simulink model "Pole_placement"  (R2023b)
settings: Solver=VariableStepAuto  StartTime=0.0  StopTime=20  MaxStep=0.05  MinStep=0.001  RelTol=1e-3
values from neighbouring files (symbols this model uses):
  A = double(A)    [Rotational_inverted_pendulum.m]
  A_uns = double(A_uns)    [Rotational_inverted_pendulum.m]
  alfa = 1e-5    (= 1e-05)    [Rotational_inverted_pendulum.m]
  B = double(B)    [Rotational_inverted_pendulum.m]
  B_uns = double(B_uns)    [Rotational_inverted_pendulum.m]
  beta = 1.295e-5    (= 1.295e-05)    [Rotational_inverted_pendulum.m]
  C = [1 0 0 0 ... (first row only)    [Rotational_inverted_pendulum.m]
  C_uns = [1 0 0 0 ... (first row only)    [Rotational_inverted_pendulum.m]
  D = [0 ... (first row only)    [Rotational_inverted_pendulum.m]
  D_uns = [0 ... (first row only)    [Rotational_inverted_pendulum.m]
  g0 = 9.81    [Rotational_inverted_pendulum.m]
  Ip = (mp*Lp^2)/12    (= 3.3282e-05)    [Rotational_inverted_pendulum.m]
  Ir = 9.6e-5    (= 9.6e-05)    [Rotational_inverted_pendulum.m]
  Ir_tot = Ir+J+J_hub    (= 0.0001006)    [Rotational_inverted_pendulum.m]
  K = 42e-3    (= 0.042)    [Rotational_inverted_pendulum.m]
  K_pp = place(A,B,P)    [Rotational_inverted_pendulum.m]
  K_pp_uns = place(A_uns,B_uns,P_uns)    [Rotational_inverted_pendulum.m]
  L_kf = lqr(A',C',Q_tilde,R_tilde)'    [Rotational_inverted_pendulum.m]
  L_kf_uns = lqr(A_uns',C_uns',Q_tilde_uns,R_tilde_uns)'    [Rotational_inverted_pendulum.m]
  L_pp = place(A',C',P_obsv)'    [Rotational_inverted_pendulum.m]
  L_pp_uns = place(A_uns',C_uns',P_obsv_uns)'    [Rotational_inverted_pendulum.m]
  La = 1.16e-3    (= 0.00116)    [Rotational_inverted_pendulum.m]
  Ld = 0.40*Lr    (= 0.034)    [Rotational_inverted_pendulum.m]
  Lp = 0.129    [Rotational_inverted_pendulum.m]
  Lr = 0.085    [Rotational_inverted_pendulum.m]
  mp = 0.024    [Rotational_inverted_pendulum.m]
  mr = 0.095    [Rotational_inverted_pendulum.m]
  phi_dot_init = 0    [Rotational_inverted_pendulum.m]
  phi_init = 0    [Rotational_inverted_pendulum.m]
  Ra = 8.4    [Rotational_inverted_pendulum.m]
  theta_dot_init = 0    [Rotational_inverted_pendulum.m]
  theta_init = 0    [Rotational_inverted_pendulum.m]
  x1_bar = double(sol.x1)    [Rotational_inverted_pendulum.m]
  x1_bar_uns = x1_bar    [Rotational_inverted_pendulum.m]
  x3_bar = 0    [Rotational_inverted_pendulum.m]
  x3_bar_uns = pi    (= 3.14159265359)    [Rotational_inverted_pendulum.m]
undefined symbols (not defined in the file or in its folder): rot_pend
libraries: simulink_extras x17
settings Model: Creator=Mark  LastModifiedBy=Mark

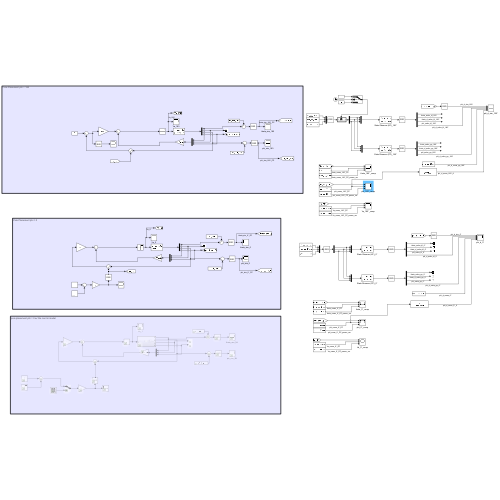
[thumbnail: Simulink's stored preview of the top-level diagram]
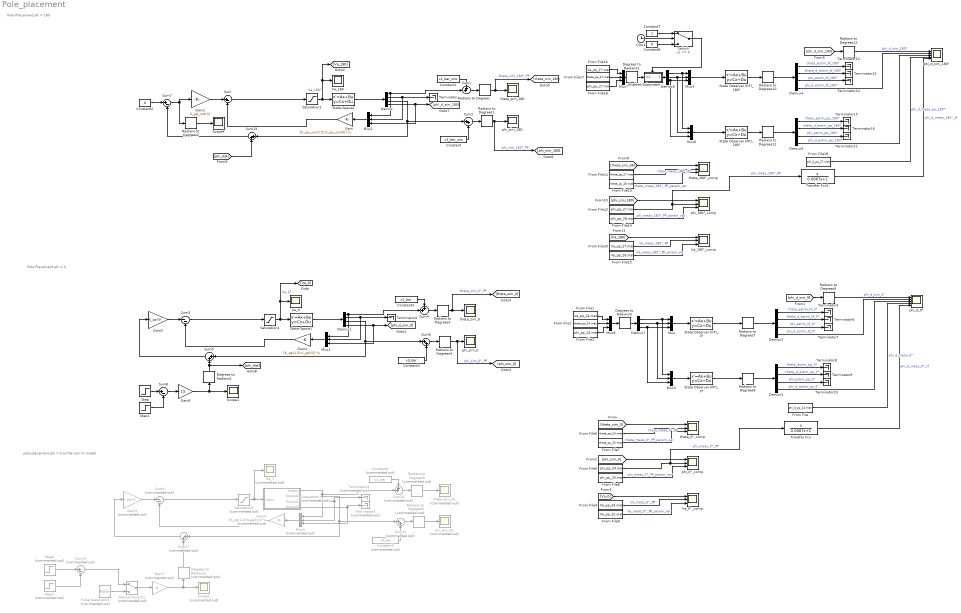
== system Pole_placement ==
  note: pole placement phi = 0 w/ the non lin model
  note: Pole Placement phi = 180
  note: Pole Placement phi = 0
  Clock : Clock
  Constant : Constant  Value=x3_bar_uns
  Constant1 : Constant  Value=x1_bar_uns
  Constant2 : Constant  Value=0
  Constant3 : Constant  Value=x3_bar
  Constant4 : Constant  Value=x1_bar
  Constant5 : Constant  Commented=on  Value=x3_bar
  Constant6 : Constant  Commented=on  Value=x1_bar
  Constant7 : Constant
  Constant8 : Constant  Value=0
  Degrees to Radians1 : simulink_extras/Transformations/Degrees to Radians
  Degrees to Radians2 : simulink_extras/Transformations/Degrees to Radians  Commented=on
  Degrees to Radians3 : simulink_extras/Transformations/Degrees to Radians
  Degrees to Radians4 : simulink_extras/Transformations/Degrees to Radians
  Demux{,1..5} (6 alike) : Demux
  Demux6 : Demux  Outputs=3
  Demux7 : Demux  Outputs=3
  Enabled Subsystem : Subsystem  TreatAsAtomicUnit=on
  From File : FromFile  FileName=phi_d_pp_24.mat  SampleTime=0
  From File1 : FromFile  FileName=Va_pp_24.mat  SampleTime=0
  From File10 : FromFile  FileName=Va_pp_27.mat  SampleTime=0
  From File11 : FromFile  FileName=theta_pp_27.mat  SampleTime=0
  From File12 : FromFile  FileName=phi_pp_27.mat  SampleTime=0
  From File13 : FromFile  FileName=theta_pp_28.mat  SampleTime=0
  From File14 : FromFile  FileName=phi_pp_28.mat  SampleTime=0
  From File15 : FromFile  FileName=Va_pp_28.mat  SampleTime=0
  From File16 : FromFile  FileName=Va_pp_27.mat  SampleTime=0
  From File17 : FromFile  FileName=theta_pp_27.mat  SampleTime=0
  From File18 : FromFile  FileName=phi_pp_27.mat  SampleTime=0
  From File19 : FromFile  FileName=phi_d_pp_27.mat  SampleTime=0
  From File2 : FromFile  FileName=theta_pp_24.mat  SampleTime=0
  From File3 : FromFile  FileName=phi_pp_24.mat  SampleTime=0
  From File4 : FromFile  FileName=Va_pp_24.mat  SampleTime=0
  From File5 : FromFile  FileName=theta_pp_24.mat  SampleTime=0
  From File6 : FromFile  FileName=phi_pp_24.mat  SampleTime=0
  From File7 : FromFile  FileName=theta_pp_25.mat  SampleTime=0
  From File8 : FromFile  FileName=phi_pp_25.mat  SampleTime=0
  From File9 : FromFile  FileName=Va_pp_25.mat  SampleTime=0
  Gain : Gain  Gain=[K_pp_uns(1:2) K_pp_uns(4)]  Multiplication=Matrix(K*u) (u vector)
  Gain1 : Gain  Gain=K_pp_uns(3)
  Gain2 : Gain  Gain=[K_pp(1:2) K_pp(4)]  Multiplication=Matrix(K*u) (u vector)
  Gain3 : Gain  Gain=K_pp(3)
  Gain4 : Gain  Commented=on  Gain=[K_pp(1:2) K_pp(4)]  Multiplication=Matrix(K*u) (u vector)
  Gain5 : Gain  Commented=on  Gain=K_pp(3)
  Gain6 : Gain  Gain=15
  Gain7 : Gain  Commented=on  Gain=5
  Manual Switch1 : ManualSwitch  Commented=on
  Mux{,1..2,4..8} (8 alike) : Mux  Inputs=3
  Mux3 : Mux  Commented=on  Inputs=3
  Pulse Generator2 : DiscretePulseGenerator  Commented=on  PulseType=Time based  Period=10000  PulseWidth=0.005  PhaseDelay=30
  Radians to Degrees{,1..4,7..12} (11 alike) : simulink_extras/Transformations/Radians to Degrees
  Radians to Degrees5 : simulink_extras/Transformations/Radians to Degrees  Commented=on
  Radians to Degrees6 : simulink_extras/Transformations/Radians to Degrees  Commented=on
  Saturation1 : Saturate  UpperLimit=10  LowerLimit=-10
  Saturation2 : Saturate  UpperLimit=10  LowerLimit=-10
  Saturation3 : Saturate  Commented=on  UpperLimit=10  LowerLimit=-10
  Scope1 : Scope
  Scope2 : Scope  Commented=on
  Scope4 : Scope
  State Observer (KF)_0° : StateSpace  A=A-L_kf*C  B=[B-L_kf*D L_kf]  C=eye(4)  D=zeros(4,3)  InitialCondition=0  ParameterTunability=Unconstrained
  State Observer (KF)_180° : StateSpace  A=A_uns-L_kf_uns*C_uns  B=[B_uns-L_kf_uns*D_uns L_kf_uns]  C=eye(4)  D=zeros(4,3)  InitialCondition=0  ParameterTunability=Unconstrained
  State Observer (PP)_0° : StateSpace  A=A-L_pp*C  B=[B-L_pp*D L_pp]  C=eye(4)  D=zeros(4,3)  InitialCondition=0
  State Observer (PP)_180° : StateSpace  A=A_uns-L_pp_uns*C_uns  B=[B_uns-L_pp_uns*D_uns L_pp_uns]  C=eye(4)  D=zeros(4,3)  InitialCondition=[0 0 0 0]
  State-Space1 : StateSpace  A=A  B=B  C=eye(4)  D=zeros(4,1)  InitialCondition=[0 0 0 0]
  State-Space2 : StateSpace  A=A_uns  B=B_uns  C=[1 0 0 0; 0 1 0 0; 0 0 1 0; 0 0 0 1]  D=[0 0 0 0]'  InitialCondition=[0 0 0 0]
  Step : Step  Time=10  SampleTime=0
  Step1 : Step  Time=10.05  SampleTime=0
  Step2 : Step  Commented=on  Time=30  SampleTime=0
  Step3 : Step  Commented=on  Time=30.05  SampleTime=0
  Subsystem1 : Subsystem  Commented=on
  Sum : Sum  Inputs=|+-
  Sum1 : Sum  Inputs=++|
  Sum10 : Sum  Commented=on  Inputs=++|
  Sum11 : Sum  Commented=on  Inputs=|++
  Sum12 : Sum  Commented=on  Inputs=|++
  Sum{2,5..6,13} (4 alike) : Sum  Inputs=|++
  Sum14 : Sum  Commented=on  Inputs=|+-
  Sum3 : Sum  Inputs=|--
  Sum4 : Sum  Inputs=++|
  Sum7 : Sum  Inputs=|+-
  Sum8 : Sum  Inputs=|+-
  Sum9 : Sum  Commented=on  Inputs=|--
  Switch : Switch  SaturateOnIntegerOverflow=off  InputSameDT=off
  Terminator{,2..3,6..16} (14 alike) : Terminator
  Terminator4 : Terminator  Commented=on
  Terminator5 : Terminator  Commented=on
  Transfer Fcn : TransferFcn  Numerator=[1 0]  Denominator=[0.0067 1]
  Transfer Fcn1 : TransferFcn  Numerator=[1 0]  Denominator=[0.0067 1]
  Va_0 : Scope
  Va_0°_comp : Scope  NumInputPorts=3
  Va_1 : Scope  Commented=on
  Va_180 : Scope
  Va_180°_comp : Scope  NumInputPorts=3
  phi_0°_comp : Scope  NumInputPorts=3
  phi_180°_comp : Scope  NumInputPorts=3
  phi_d_0° : Scope  NumInputPorts=5
  phi_d_sim_180° : Scope  NumInputPorts=5
  phi_sim_0 : Scope
  phi_sim_180 : Scope
  phi_sim_NL : Scope  Commented=on
  theta_0°_comp : Scope  NumInputPorts=3
  theta_180°_comp : Scope  NumInputPorts=3
  theta_sim_0 : Scope
  theta_sim_180 : Scope
  theta_sim_NL : Scope  Commented=on
  wires:
  Demux/1 -> Mux1/1, Sum1/2
  Radians to Degrees/1 -> [theta_sim_180], theta_sim_180/1  "theta_sim_180°_PP"
  State-Space2/1 -> Demux/1
  Gain/1 -> Sum/2
  Saturation1/1 -> [Va_180], Va_180/1, State-Space2/1  "Va_180°"
  Demux/3 -> Sum2/1, Sum13/1
  Gain1/1 -> Sum/1
  Demux/2 -> Mux1/2, Terminator/1
  Demux/4 -> [phi_d_sim_180], Mux1/3
  Sum/1 -> Saturation1/1
  Radians to Degrees1/1 -> [phi_sim_180], phi_sim_180/1  "phi_sim_180°_PP"
  Sum2/1 -> Radians to Degrees1/1
  Sum1/1 -> Radians to Degrees/1
  Constant/1 -> Sum2/2
  Constant1/1 -> Sum1/1
  Mux1/1 -> Gain/1
  Sum13/1 -> Sum7/2
  Sum7/1 -> Gain1/1, Radians to Degrees2/1
  Radians to Degrees2/1 -> Scope4/1
  [phi_dist] -> Sum13/2
  Constant2/1 -> Sum7/1
  Radians to Degrees4/1 -> [phi_sim_0], phi_sim_0/1  "phi_sim_0°_PP"
  Sum5/1 -> Gain3/1
  Gain6/1 -> Scope1/1, Degrees to Radians1/1
  Step/1 -> Sum8/1
  Demux1/1 -> Mux2/1, Sum4/2
  State-Space1/1 -> Demux1/1
  Sum8/1 -> Gain6/1
  Constant3/1 -> Sum6/2
  Mux2/1 -> Gain2/1
  Saturation2/1 -> [Va_0], Va_0/1, State-Space1/1  "Va_0°"
  Sum3/1 -> Saturation2/1
  Demux1/2 -> Mux2/2, Terminator2/1
  Step1/1 -> Sum8/2
  Radians to Degrees3/1 -> [theta_sim_0], theta_sim_0/1  "theta_sim_0°_PP"
  Gain2/1 -> Sum3/2
  Demux1/4 -> [phi_d_sim_0], Mux2/3
  Sum6/1 -> Radians to Degrees4/1
  Demux1/3 -> Sum6/1, Sum5/1
  Sum4/1 -> Radians to Degrees3/1
  Gain3/1 -> Sum3/1
  Constant4/1 -> Sum4/1
  Degrees to Radians1/1 -> [phi_dist], Sum5/2
  Saturation3/1 -> Subsystem1/1(Input), Va_1/1
  Subsystem1/1(Output) -> Mux3/1, Sum10/2
  Step2/1 -> Sum14/1
  Pulse Generator2/1 -> Manual Switch1/2
  Gain7/1 -> Scope2/1, Degrees to Radians2/1
  Radians to Degrees6/1 -> phi_sim_NL/1
  Sum11/1 -> Gain5/1
  Constant5/1 -> Sum12/2
  Sum14/1 -> Manual Switch1/1
  Subsystem1/2(Output2) -> Sum12/1, Sum11/1
  Sum12/1 -> Radians to Degrees6/1
  Subsystem1/4(Output3) -> Terminator5/1, Mux3/3
  Mux3/1 -> Gain4/1
  Constant6/1 -> Sum10/1
  Degrees to Radians2/1 -> Sum11/2
  Gain5/1 -> Sum9/1
  Gain4/1 -> Sum9/2
  Manual Switch1/1 -> Gain7/1
  Sum10/1 -> Radians to Degrees5/1
  Step3/1 -> Sum14/2
  Radians to Degrees5/1 -> theta_sim_NL/1
  Subsystem1/3(Output1) -> Terminator4/1, Mux3/2
  Sum9/1 -> Saturation3/1
  Demux2/2 -> Terminator6/1  "theta_d_estim_kf_0°"
  State Observer (PP)_0°/1 -> Radians to Degrees8/1
  Demux3/4 -> phi_d_0°/3  "phi_d_estim_pp_0°"
  Demux3/2 -> Terminator9/1  "theta_d_estim_pp_0°"
  Mux4/1 -> State Observer (PP)_0°/1
  Demux2/3 -> Terminator7/1  "phi_estim_kf_0°"
  Radians to Degrees8/1 -> Demux3/1
  Demux3/3 -> Terminator10/1  "phi_estim_pp_0°"
  Radians to Degrees7/1 -> Demux2/1
  Mux/1 -> State Observer (KF)_0°/1
  Demux2/4 -> phi_d_0°/2  "phi_d_estim_kf_0°"
  State Observer (KF)_0°/1 -> Radians to Degrees7/1
  Demux2/1 -> Terminator3/1  "theta_estim_kf_0°"
  Demux3/1 -> Terminator8/1  "theta_estim_pp_0°"
  Demux7/1 -> Mux4/1, Mux/1
  Demux7/2 -> Mux4/2, Mux/2
  Demux7/3 -> Mux4/3, Mux/3
  [phi_d_sim_0] -> Radians to Degrees9/1
  Radians to Degrees9/1 -> phi_d_0°/1  "phi_d_sim_0°"
  Radians to Degrees12/1 -> phi_d_sim_180°/1  "phi_d_sim_180°"
  Demux5/1 -> Terminator15/1  "theta_estim_pp_180°"
  Radians to Degrees11/1 -> Demux5/1
  State Observer (KF)_180°/1 -> Radians to Degrees10/1
  Radians to Degrees10/1 -> Demux4/1
  Demux6/3 -> Mux6/3, Mux5/3
  Demux5/2 -> Terminator16/1  "theta_d_estim_pp_180°"
  Demux4/4 -> phi_d_sim_180°/2  "phi_d_estim_kf_180°"
  [phi_d_sim_180] -> Radians to Degrees12/1
  Demux6/2 -> Mux6/2, Mux5/2
  Demux5/4 -> phi_d_sim_180°/3  "phi_d_estim_pp_180°"
  Demux4/1 -> Terminator12/1  "theta_estim_kf_180°"
  Demux5/3 -> Terminator11/1  "phi_estim_pp_180°"
  Demux6/1 -> Mux6/1, Mux5/1
  Demux4/2 -> Terminator13/1  "theta_d_estim_kf_180°"
  State Observer (PP)_180°/1 -> Radians to Degrees11/1
  Demux4/3 -> Terminator14/1  "phi_estim_kf_180°"
  From File/1 -> phi_d_0°/4  "phi_d_meas_0°"
  [theta_sim_0] -> theta_0°_comp/1
  From File5/1 -> theta_0°_comp/2  "theta_meas_0°_PP"
  [phi_sim_0] -> phi_0°_comp/1
  From File6/1 -> Transfer Fcn/1, phi_0°_comp/2  "phi_meas_0°_PP"
  [Va_0] -> Va_0°_comp/1
  From File4/1 -> Va_0°_comp/2  "Va_meas_0°_PP"
  From File16/1 -> Mux7/1
  From File17/1 -> Mux7/2
  Mux7/1 -> Degrees to Radians3/1
  Degrees to Radians3/1 -> Enabled Subsystem/1(In1)
  Degrees to Radians4/1 -> Demux7/1
  Mux8/1 -> Degrees to Radians4/1
  From File1/1 -> Mux8/1
  From File2/1 -> Mux8/2
  From File3/1 -> Mux8/3
  From File7/1 -> theta_0°_comp/3  "theta_meas_0°_PP_param_var"
  From File8/1 -> phi_0°_comp/3  "phi_meas_0°_PP_param_var"
  From File9/1 -> Va_0°_comp/3  "Va_meas_0°_PP_param_var"
  From File11/1 -> theta_180°_comp/2  "theta_meas_180°_PP"
  [theta_sim_180] -> theta_180°_comp/1
  [Va_180] -> Va_180°_comp/1
  From File13/1 -> theta_180°_comp/3  "theta_meas_180°_PP_param_var"
  [phi_sim_180] -> phi_180°_comp/1
  From File10/1 -> Va_180°_comp/2  "Va_meas_180°_PP"
  From File15/1 -> Va_180°_comp/3  "Va_meas_180°_PP_param_var"
  From File12/1 -> Transfer Fcn1/1, phi_180°_comp/2  "phi_meas_180°_PP"
  From File14/1 -> phi_180°_comp/3  "phi_meas_180°_PP_param_var"
  From File19/1 -> phi_d_sim_180°/4  "phi_d_meas_pp_180°"
  From File18/1 -> Mux7/3
  Constant7/1 -> Switch/1
  Constant8/1 -> Switch/3
  Clock/1 -> Switch/2
  Mux5/1 -> State Observer (KF)_180°/1
  Mux6/1 -> State Observer (PP)_180°/1
  Enabled Subsystem/1(Out1) -> Demux6/1
  Switch/1 -> Enabled Subsystem/Enable
  Transfer Fcn/1 -> phi_d_0°/5  "phi_d_meas_0°_tf"
  Transfer Fcn1/1 -> phi_d_sim_180°/5  "phi_d_meas_180°_tf"

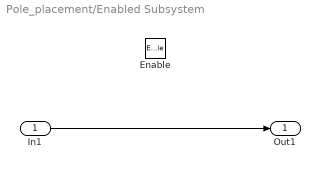
== system Pole_placement/Enabled Subsystem ==
  In1 : Inport
  Enable : EnablePort
  Out1 : Outport
  wires:
  In1/1 -> Out1/1

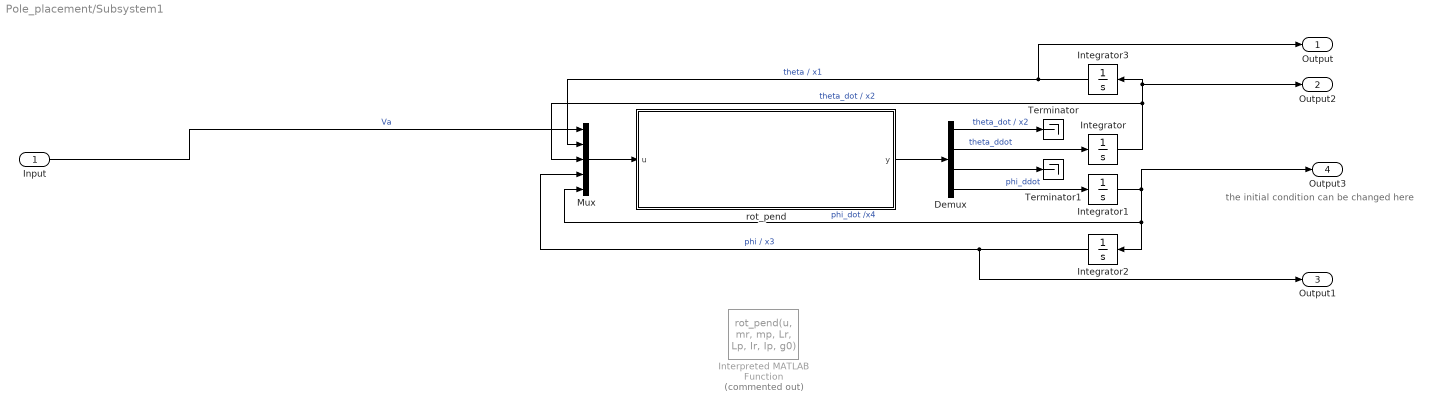
== system Pole_placement/Subsystem1 ==
  note: the initial condition can be changed here
  Input : Inport
  Demux : Demux
  Integrator : Integrator  InitialCondition=theta_dot_init
  Integrator1 : Integrator  InitialCondition=phi_dot_init
  Integrator2 : Integrator  InitialCondition=phi_init
  Integrator3 : Integrator  InitialCondition=theta_init
  Interpreted MATLAB Function : MATLABFcn  Commented=on  MATLABFcn=rot_pend(u, mr, mp, Lr, Lp, Ir, Ip, g0)  OutputDimensions=4  OutputSignalType=real
  Mux : Mux  Inputs=5
  Terminator : Terminator
  Terminator1 : Terminator
  rot_pend : Subsystem
  Output : Outport
  Output2 : Outport  Port=2
  Output1 : Outport  Port=3
  Output3 : Outport  Port=4
  wires:
  Integrator2/1 -> Output1/1, Mux/4  "phi / x3"
  Integrator/1 -> Output2/1, Integrator3/1, Mux/3  "theta_dot / x2"
  Mux/1 -> rot_pend/1(u)
  rot_pend/1(y) -> Demux/1
  Integrator1/1 -> Mux/5, Integrator2/1, Output3/1  "phi_dot /x4"
  Integrator3/1 -> Mux/2, Output/1  "theta / x1"
  Demux/4 -> Integrator1/1  "phi_ddot"
  Demux/2 -> Integrator/1  "theta_ddot"
  Demux/1 -> Terminator/1  "theta_dot / x2"
  Demux/3 -> Terminator1/1
  Input/1 -> Mux/1  "Va"

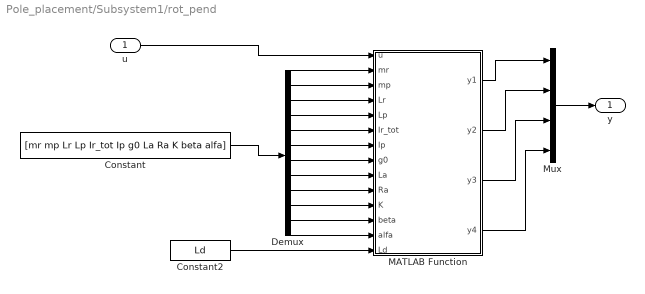
== system Pole_placement/Subsystem1/rot_pend ==
  u : Inport
  Constant : Constant  Value=[mr mp Lr Lp Ir_tot Ip g0 La Ra K beta alfa]  VectorParams1D=off
  Constant2 : Constant  Value=Ld
  Demux : Demux  Outputs=12
  MATLAB Function : MATLAB Function  TreatAsAtomicUnit=on
  Mux : Mux
  y : Outport
  wires:
  Demux/3 -> MATLAB Function/4(Lr)
  Demux/5 -> MATLAB Function/6(Ir_tot)
  Demux/4 -> MATLAB Function/5(Lp)
  Demux/7 -> MATLAB Function/8(g0)
  Demux/2 -> MATLAB Function/3(mp)
  Demux/6 -> MATLAB Function/7(Ip)
  Demux/1 -> MATLAB Function/2(mr)
  u/1 -> MATLAB Function/1(u)
  Constant/1 -> Demux/1
  MATLAB Function/1(y1) -> Mux/1
  MATLAB Function/2(y2) -> Mux/2
  MATLAB Function/3(y3) -> Mux/3
  MATLAB Function/4(y4) -> Mux/4
  Mux/1 -> y/1
  Demux/8 -> MATLAB Function/9(La)
  Demux/9 -> MATLAB Function/10(Ra)
  Demux/10 -> MATLAB Function/11(K)
  Demux/11 -> MATLAB Function/12(beta)
  Constant2/1 -> MATLAB Function/14(Ld)
  Demux/12 -> MATLAB Function/13(alfa)

== matlab function Pole_placement/Subsystem1/rot_pend/MATLAB Function ==
  data: u input; y1 output; mr input; mp input; Lr input; Lp input; Ir_tot input; Ip input; g0 input; La input; Ra input; y2 output; y3 output; y4 output; K input; beta input; alfa input; Ld input
function [y1,y2,y3,y4] = rot_pend(u, mr, mp, Lr, Lp, Ir_tot, Ip, g0,La, Ra, K, beta,alfa, Ld)
%UNTITLED Summary of this function goes here
%   Detailed explanation goes here
% u(1) = Va
x1 = u(2) ; % theta
x2 = u(3) ; % theta_dot
x3 = u(4) ; % phi
x4 = u(5) ; % phi_dot

H = [(mp*(Lr^2+((Lp/2)^2*(sin(x3))^2)))+Ir_tot            -mp*Lr*Lp*cos(x3)/2;
                     -mp*Lr*Lp*cos(x3)/2                              (mp*(Lp/2)^2)+Ip] ;

Q = [mp*(Lp/2)^2*sin(x3)*cos(x3)*x4+beta                     (mp*(Lp/2)^2*sin(x3)*cos(x3)*x2)-(mp*Lr*(Lp/2)*sin(x3)*x4);
     -mp*(Lp/2)^2*sin(x3)*cos(x3)*x2                                                   alfa                                   ] ;

g = [           0     ;
     mp*g0*(Lp/2)*sin(x3)] ;
%(K*u(1)/Ra)-(K^2*x2/Ra)
tau = [(K/Ra)*(u(1)-(K*x2)) ;
       0 ] ;

if (x1>=0.1745 | x1<=-0.1745)       % 0.08727rad = 5deg
     kt = 0.03 ;                    % 0.1745rad = 10deg
     kc = 10e-3 ;
else                               % 0.349rad = 20deg
    kt = 0 ;
    kc = 3.5e-3 ;
end
% if (x2>=2.618 | x2<=-2.618)       % 3.49rad/s = 200deg/s
%                                 % 2.618rad/s = 150deg/s
%     kc = 10e-3 ;
% else                               
% 
%     kc = 4.8e-3 ;
% end


Tr_theta = ((kt*x1)+(kc*x2))*Ld ;
q_ddot = H\[tau - Q*[x2 x4]' - g - [Tr_theta 0]' ] ;



y1 = x2 ;
y2 = q_ddot(1) ;
y3 = x4 ;
y4 = q_ddot(2) ;


%Ir+mr*(Lr/2)^2)
